simulink model "GasTurbine_PolyCompare_R3_Poly2FF"  (Simulink 9.2)
settings: Solver=ode4  StartTime=0.0  StopTime=MWS.in.SimTime  FixedStep=MWS.Solve.T  RelTol=1e-3  EnableMultiTasking=on
PreLoadFcn:
  | tmats_r3_poly2_setup;
values from neighbouring files (symbols this model uses):
  DOB = DOB0; DOB.gain=gains(j);DOB.mode=modes(j);DOB.fc=fcs(j)    [run_tmats_dob_study.m]
  MWS = tmats_gpt_setup()    [run_tmats_gpt.m]
undefined symbols (not defined in the file or in its folder): PTO, stripchar_TMATS, VF
libraries: Lib_Cntrl_FirstOrderSensor_TMATS x1, simulink x1, Lib_Turbo_Ambient_TMATS x1, Lib_Turbo_Burner_TMATS x1, Lib_Turbo_Compressor_TMATS x1, Lib_Turbo_Duct_TMATS x1, Lib_Turbo_Inlet_TMATS x1, Lib_Turbo_Nozzle_TMATS x1, Lib_Turbo_Shaft_TMATS x1, Lib_Turbo_Turbine_TMATS x1, Lib_Solve_IterNRSolverJC_TMATS x1, Lib_Solve_ModelSource_TMATS x1
Description:
  | 120 s speed-ramp and ambient cycle. See the cycle study usage notes.
settings Model: Creator=jwchapm2  LastModifiedBy=volka
settings DataIOCC: SignalLoggingSaveFormat=Dataset  SignalLoggingName=SimulationOutput
settings OptimizationCC: BlockReduction=off  DefaultParameterBehavior=Inlined  BufferReuse=off  ExpressionDepthLimit=2147483647
settings DebuggingCC: AlgebraicLoopMsg=error  SolverPrmCheckMsg=warning  FcnCallInpInsideContextMsg=error
settings GRTTargetCC: CombineOutputUpdateFcns=on  GRTInterface=off

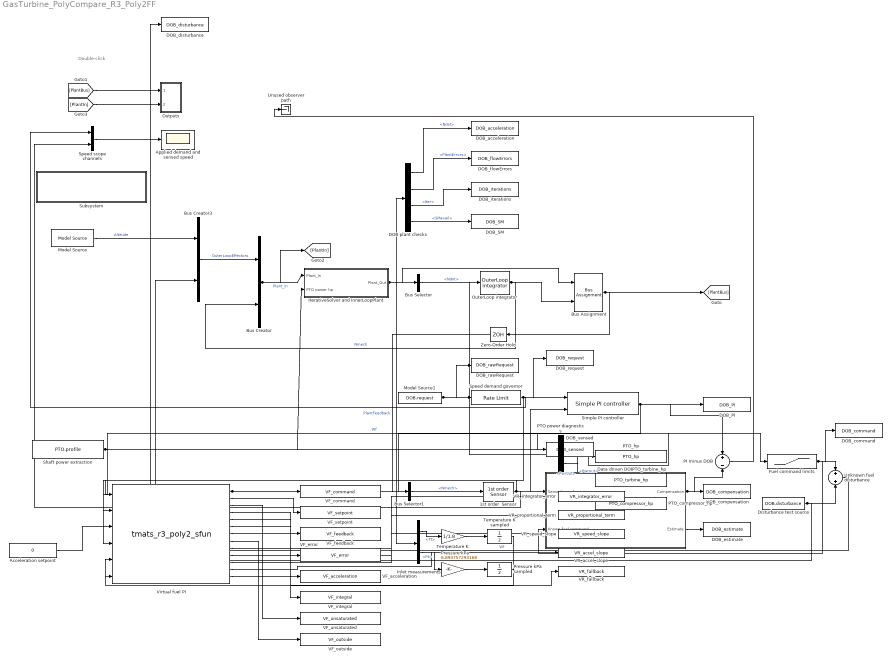
== system GasTurbine_PolyCompare_R3_Poly2FF ==
  note: Double-click
  1st order  Sensor : Lib_Cntrl_FirstOrderSensor_TMATS/1st order  Sensor  IC_M=MWS.Solve.N_IC  Sen_Max_M=20000  Sen_Min_M=0  Gain_M=1  Tau_M=0.05  GN_EN_M=off  GN_NST_M=MWS.Solve.T  GN_C_M=1  GN_MinNoise_M=0.3  F_Gain_M=1  F_Drift_M=0
  Acceleration setpoint : Constant  Value=0
  Applied demand and sensed speed : Scope
  Bus Assignment : BusAssignment  AssignedSignals=PlantBus.Nmech
  Bus Creator : BusCreator  Inputs=2
  Bus Creator3 : BusCreator  Inputs=2
  Bus Selector : BusSelector  OutputSignals=PlantBus.Ndot
  Bus Selector1 : BusSelector  OutputSignals=PlantBus.Nmech
  DOB plant checks : BusSelector  OutputSignals=PlantBus.Ndot,PlantErrors,PlantBus.Iter,PlantBus.C_Data.SMavail
  DOB_PI : ToWorkspace  VariableName=DOB_PI  SaveFormat=Timeseries  SampleTime=-1
  DOB_SM : ToWorkspace  VariableName=DOB_SM  SaveFormat=Timeseries  SampleTime=-1
  DOB_acceleration : ToWorkspace  VariableName=DOB_acceleration  SaveFormat=Timeseries  SampleTime=-1
  DOB_command : ToWorkspace  VariableName=DOB_command  SaveFormat=Timeseries  SampleTime=-1
  DOB_compensation : ToWorkspace  VariableName=DOB_compensation  SaveFormat=Timeseries  SampleTime=-1
  DOB_disturbance : ToWorkspace  VariableName=DOB_disturbance  SaveFormat=Timeseries  SampleTime=-1
  DOB_estimate : ToWorkspace  VariableName=DOB_estimate  SaveFormat=Timeseries  SampleTime=-1
  DOB_flowErrors : ToWorkspace  VariableName=DOB_flowErrors  SaveFormat=Timeseries  SampleTime=-1
  DOB_iterations : ToWorkspace  VariableName=DOB_iterations  SaveFormat=Timeseries  SampleTime=-1
  DOB_rawRequest : ToWorkspace  VariableName=DOB_rawRequest  SaveFormat=Timeseries  SampleTime=-1
  DOB_request : ToWorkspace  VariableName=DOB_request  SaveFormat=Timeseries  SampleTime=-1
  DOB_sensed : ToWorkspace  VariableName=DOB_sensed  SaveFormat=Timeseries  SampleTime=-1
  Data driven DOB : Subsystem
  Disturbance test source : FromWorkspace  VariableName=DOB.disturbance  SampleTime=DOB.Ts  Interpolate=off  OutputAfterFinalValue=Holding final value
  Fuel command limits : Saturate  UpperLimit=DOB.fuelMax  LowerLimit=DOB.fuelMin
  Inlet measurements : BusSelector  OutputSignals=PlantBus.s2.Tt,PlantBus.s2.Pt
  IterativeSolver and InnerLoopPlant : Subsystem
  Model Source : Lib_Solve_ModelSource_TMATS/Model Source  T_vec_M=MWS.in.t_vec  input_array_M=MWS.in.Alt
  Model Source1 : FromWorkspace  VariableName=DOB.request  SampleTime=DOB.Ts  Interpolate=off  OutputAfterFinalValue=Holding final value
  OuterLoop integrator : Lib_Solve_OuterLoopIntegrator_TMATS/OuterLoop integrator  OL_IC_M=MWS.Solve.N_IC
  Outputs : Subsystem
  PI minus DOB : Sum  Inputs=+-
  PTO power diagnostics : BusSelector  OutputSignals=PlantBus.T_Data.Pwrout,PlantBus.C_Data.Pwrout
  PTO_compressor_hp : ToWorkspace  VariableName=PTO_compressor_hp  SaveFormat=Timeseries  SampleTime=-1
  PTO_hp : ToWorkspace  VariableName=PTO_hp  SaveFormat=Timeseries  SampleTime=-1
  PTO_turbine_hp : ToWorkspace  VariableName=PTO_turbine_hp  SaveFormat=Timeseries  SampleTime=-1
  Pressure kPa : Gain  Gain=6.894757293168
  Pressure kPa sampled : UnitDelay  InitialCondition=99.298  SampleTime=VF.Ts
  Shaft power extraction : FromWorkspace  VariableName=PTO.profile  SampleTime=PTO.Ts  Interpolate=off  OutputAfterFinalValue=Holding final value
  Simple PI controller : Lib_Cntrl_SimplePIcontroller_TMATS/Simple PI controller  Kp_M=0.05/2  Ki_M=0.1/2  PI_IC_M=3
  Speed demand governor : RateLimiter  RisingSlewLimit=DOB.rate  FallingSlewLimit=-DOB.rate  SampleTimeMode=inherited  InitialCondition=10000
  Speed scope channels : Mux  Inputs=2
  Subsystem : Subsystem
      settings: OpenFcn=run('PlotDynData.m')
      mask Display: fprintf('Plot Outputs')
  Temperature K : Gain  Gain=1/1.8
  Temperature K sampled : UnitDelay  InitialCondition=288.15  SampleTime=VF.Ts
  Unknown fuel disturbance : Sum
  Unused observer path : Terminator
  VF_acceleration : ToWorkspace  VariableName=VF_acceleration  SaveFormat=Timeseries  SampleTime=-1
  VF_command : ToWorkspace  VariableName=VF_command  SaveFormat=Timeseries  SampleTime=-1
  VF_error : ToWorkspace  VariableName=VF_error  SaveFormat=Timeseries  SampleTime=-1
  VF_feedback : ToWorkspace  VariableName=VF_feedback  SaveFormat=Timeseries  SampleTime=-1
  VF_integral : ToWorkspace  VariableName=VF_integral  SaveFormat=Timeseries  SampleTime=-1
  VF_outside : ToWorkspace  VariableName=VF_outside  SaveFormat=Timeseries  SampleTime=-1
  VF_setpoint : ToWorkspace  VariableName=VF_setpoint  SaveFormat=Timeseries  SampleTime=-1
  VF_unsaturated : ToWorkspace  VariableName=VF_unsaturated  SaveFormat=Timeseries  SampleTime=-1
  VR_accel_slope : ToWorkspace  VariableName=VR_accel_slope  SaveFormat=Timeseries  SampleTime=-1
  VR_fallback : ToWorkspace  VariableName=VR_fallback  SaveFormat=Timeseries  SampleTime=-1
  VR_integrator_error : ToWorkspace  VariableName=VR_integrator_error  SaveFormat=Timeseries  SampleTime=-1
  VR_proportional_term : ToWorkspace  VariableName=VR_proportional_term  SaveFormat=Timeseries  SampleTime=-1
  VR_speed_slope : ToWorkspace  VariableName=VR_speed_slope  SaveFormat=Timeseries  SampleTime=-1
  Virtual fuel PI : M-S-Function  FunctionName=tmats_r3_poly2_sfun  Parameters=VF
  Zero-Order Hold : ZeroOrderHold  SampleTime=MWS.Solve.T
  wires:
  Data driven DOB/1(Compensation) -> PI minus DOB/2, DOB_compensation/1
  Bus Creator/1 -> [PlantIn], IterativeSolver and InnerLoopPlant/1(Plant_In)  "Plant_In"
  1st order  Sensor/1 -> Simple PI controller/2, Data driven DOB/1(Sensed speed), DOB_sensed/1, Speed scope channels/2, Virtual fuel PI/1
  OuterLoop integrator/1 -> Bus Creator/2, Bus Assignment/2  "Nmech"
  IterativeSolver and InnerLoopPlant/1(Plant_Out) -> Bus Assignment/1, Bus Selector/1, DOB plant checks/1, PTO power diagnostics/1, Inlet measurements/1
  Disturbance test source/1 -> Unknown fuel disturbance/2, DOB_disturbance/1
  Model Source1/1 -> Speed demand governor/1, DOB_rawRequest/1
  Fuel command limits/1 -> Unknown fuel disturbance/1, Data driven DOB/2(Known fuel command), DOB_command/1
  Simple PI controller/1 -> PI minus DOB/1, DOB_PI/1, Virtual fuel PI/4  "Wf"
  Speed demand governor/1 -> Simple PI controller/1, DOB_request/1, Speed scope channels/1, Virtual fuel PI/2
  Bus Assignment/1 -> [PlantBus], Zero-Order Hold/1
  Speed scope channels/1 -> Applied demand and sensed speed/1
  [PlantIn] -> Outputs/2(PlantIn)
  Data driven DOB/2(Estimate) -> DOB_estimate/1
  DOB plant checks/1 -> DOB_acceleration/1  "<Ndot>"
  DOB plant checks/2 -> DOB_flowErrors/1  "<PlantErrors>"
  Bus Creator3/1 -> Bus Creator/1  "OuterLoopEffectors"
  DOB plant checks/3 -> DOB_iterations/1  "<Iter>"
  DOB plant checks/4 -> DOB_SM/1  "<SMavail>"
  Unknown fuel disturbance/1 -> Bus Creator3/2  "Wf"
  [PlantBus] -> Outputs/1(PlantOut)
  Model Source/1 -> Bus Creator3/1  "Altitude"
  Bus Selector1/1 -> 1st order  Sensor/1  "<Nmech>"
  Bus Selector/1 -> OuterLoop integrator/1  "<Ndot>"
  Zero-Order Hold/1 -> Bus Selector1/1  "PlantFeedback"
  Shaft power extraction/1 -> IterativeSolver and InnerLoopPlant/2(PTO power hp), PTO_hp/1
  PTO power diagnostics/1 -> PTO_turbine_hp/1  "<Pwrout>"
  PTO power diagnostics/2 -> PTO_compressor_hp/1  "<Pwrout>"
  Acceleration setpoint/1 -> Virtual fuel PI/3
  PI minus DOB/1 -> Unused observer path/1
  Virtual fuel PI/1 -> Fuel command limits/1, VF_command/1
  Virtual fuel PI/2 -> VF_setpoint/1
  Virtual fuel PI/3 -> VF_feedback/1
  Virtual fuel PI/4 -> VF_error/1
  Virtual fuel PI/5 -> VF_acceleration/1
  Virtual fuel PI/6 -> VF_integral/1
  Virtual fuel PI/7 -> VF_unsaturated/1
  Virtual fuel PI/8 -> VF_outside/1
  Inlet measurements/1 -> Temperature K/1  "<Tt>"
  Temperature K/1 -> Temperature K sampled/1
  Temperature K sampled/1 -> Virtual fuel PI/5
  Inlet measurements/2 -> Pressure kPa/1  "<Pt>"
  Pressure kPa/1 -> Pressure kPa sampled/1
  Pressure kPa sampled/1 -> Virtual fuel PI/6
  Virtual fuel PI/9 -> VR_integrator_error/1
  Virtual fuel PI/10 -> VR_proportional_term/1
  Virtual fuel PI/11 -> VR_speed_slope/1
  Virtual fuel PI/12 -> VR_accel_slope/1
  Virtual fuel PI/13 -> VR_fallback/1

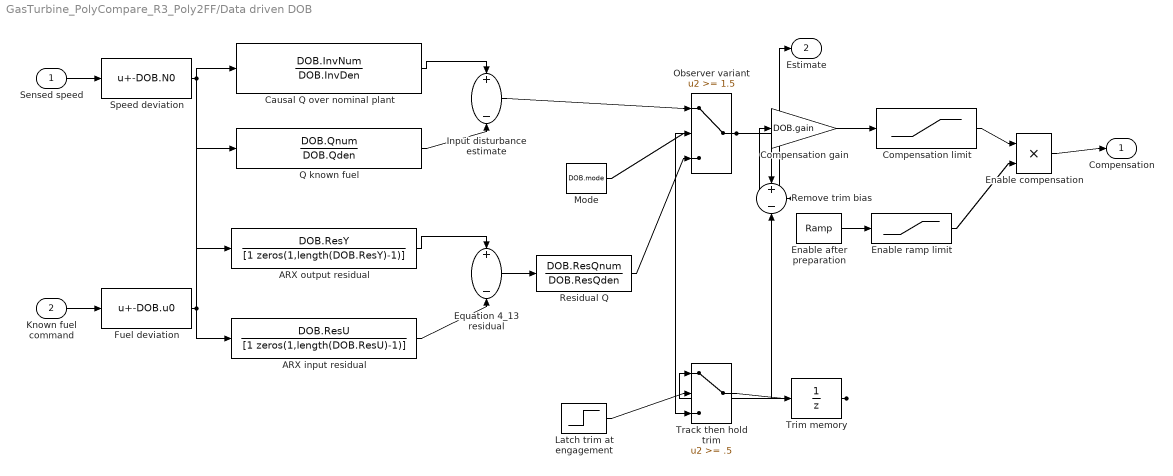
== system GasTurbine_PolyCompare_R3_Poly2FF/Data driven DOB ==
  Sensed speed : Inport
  Known fuel command : Inport  Port=2
  ARX input residual : DiscreteTransferFcn  Numerator=DOB.ResU  Denominator=[1 zeros(1,length(DOB.ResU)-1)]  SampleTime=DOB.Ts
  ARX output residual : DiscreteTransferFcn  Numerator=DOB.ResY  Denominator=[1 zeros(1,length(DOB.ResY)-1)]  SampleTime=DOB.Ts
  Causal Q over nominal plant : DiscreteTransferFcn  Numerator=DOB.InvNum  Denominator=DOB.InvDen  SampleTime=DOB.Ts
  Compensation gain : Gain  Gain=DOB.gain
  Compensation limit : Saturate  UpperLimit=DOB.compLimit  LowerLimit=-DOB.compLimit
  Enable after preparation : simulink/Sources/Ramp  slope=1/DOB.enableTime  start=DOB.start  InitialOutput=0
  Enable compensation : Product
  Enable ramp limit : Saturate  UpperLimit=1  LowerLimit=0
  Equation 4_13 residual : Sum  Inputs=+-
  Fuel deviation : Bias  Bias=-DOB.u0
  Input disturbance estimate : Sum  Inputs=+-
  Latch trim at engagement : Step  Time=DOB.start  SampleTime=DOB.Ts
  Mode : Constant  Value=DOB.mode
  Observer variant : Switch  Threshold=1.5
  Q known fuel : DiscreteTransferFcn  Numerator=DOB.Qnum  Denominator=DOB.Qden  SampleTime=DOB.Ts
  Remove trim bias : Sum  Inputs=+-
  Residual Q : DiscreteTransferFcn  Numerator=DOB.ResQnum  Denominator=DOB.ResQden  SampleTime=DOB.Ts
  Speed deviation : Bias  Bias=-DOB.N0
  Track then hold trim : Switch  Threshold=.5
  Trim memory : UnitDelay  SampleTime=DOB.Ts
  Compensation : Outport
  Estimate : Outport  Port=2
  wires:
  Sensed speed/1 -> Speed deviation/1
  Known fuel command/1 -> Fuel deviation/1
  Speed deviation/1 -> Causal Q over nominal plant/1, ARX output residual/1
  Fuel deviation/1 -> Q known fuel/1, ARX input residual/1
  Causal Q over nominal plant/1 -> Input disturbance estimate/1
  Q known fuel/1 -> Input disturbance estimate/2
  ARX output residual/1 -> Equation 4_13 residual/1
  ARX input residual/1 -> Equation 4_13 residual/2
  Equation 4_13 residual/1 -> Residual Q/1
  Input disturbance estimate/1 -> Observer variant/1
  Mode/1 -> Observer variant/2
  Residual Q/1 -> Observer variant/3
  Trim memory/1 -> Track then hold trim/1, Remove trim bias/2
  Latch trim at engagement/1 -> Track then hold trim/2
  Observer variant/1 -> Track then hold trim/3, Remove trim bias/1
  Track then hold trim/1 -> Trim memory/1
  Remove trim bias/1 -> Compensation gain/1, Estimate/1
  Compensation gain/1 -> Compensation limit/1
  Enable after preparation/1 -> Enable ramp limit/1
  Compensation limit/1 -> Enable compensation/1
  Enable ramp limit/1 -> Enable compensation/2
  Enable compensation/1 -> Compensation/1

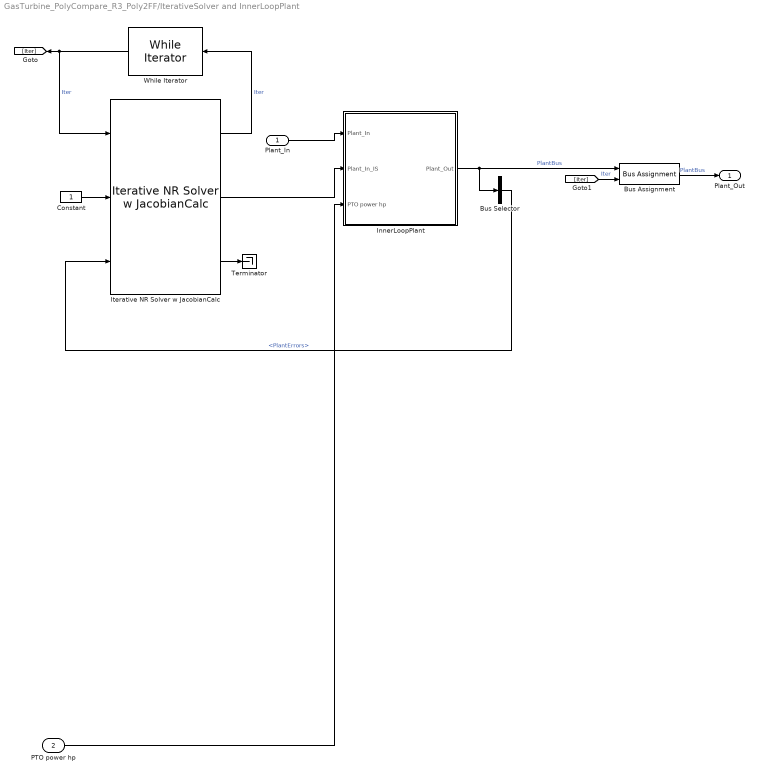
== system GasTurbine_PolyCompare_R3_Poly2FF/IterativeSolver and InnerLoopPlant ==
  Plant_In : Inport
  PTO power hp : Inport  Port=2
  Bus Assignment : BusAssignment  AssignedSignals=PlantBus.Iter
  Bus Selector : BusSelector  OutputSignals=PlantErrors
  Constant : Constant
  InnerLoopPlant : Subsystem
  Iterative NR Solver w JacobianCalc : Lib_Solve_IterNRSolverJC_TMATS/Iterative NR Solver w JacobianCalc  SJac_Per_M=MWS.Solve.J_Calc_Per  SNR_IC_M=MWS.Solve.NR_IC  SNR_DX_M=MWS.Solve.NR_dx  SNR_Mx_M=100000  SNR_Mn_M=0.0001  SJacobianAttempts_M=MWS.Solve.NR_Jac_Re  Cond_Limits_M=MWS.Solve.C_Lim
  Terminator : Terminator
  While Iterator : WhileIterator  MaxIters=MWS.Solve.Max_Iter  WhileBlockType=do-while  ShowIterationPort=on
  Plant_Out : Outport
  wires:
  Plant_In/1 -> InnerLoopPlant/1(Plant_In)
  Bus Selector/1 -> Iterative NR Solver w JacobianCalc/3  "<PlantErrors>"
  While Iterator/1 -> [Iter], Iterative NR Solver w JacobianCalc/1  "Iter"
  InnerLoopPlant/1(Plant_Out) -> Bus Assignment/1, Bus Selector/1  "PlantBus"
  Iterative NR Solver w JacobianCalc/2 -> InnerLoopPlant/2(Plant_In_IS)
  Iterative NR Solver w JacobianCalc/1 -> While Iterator/1  "Iter"
  Iterative NR Solver w JacobianCalc/3 -> Terminator/1
  Constant/1 -> Iterative NR Solver w JacobianCalc/2
  [Iter] -> Bus Assignment/2  "Iter"
  Bus Assignment/1 -> Plant_Out/1  "PlantBus"
  PTO power hp/1 -> InnerLoopPlant/3(PTO power hp)

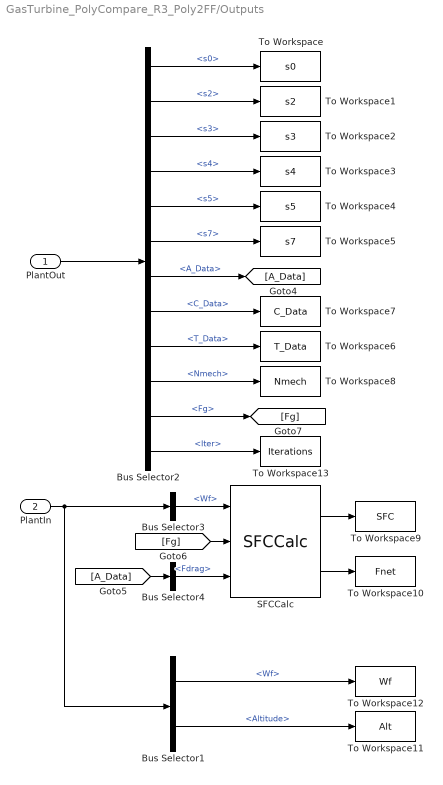
== system GasTurbine_PolyCompare_R3_Poly2FF/Outputs ==
  PlantOut : Inport
  PlantIn : Inport  Port=2
  Bus Selector1 : BusSelector  OutputSignals=OuterLoopEffectors.Wf,OuterLoopEffectors.Altitude
  Bus Selector2 : BusSelector  OutputSignals=PlantBus.s0,PlantBus.s2,PlantBus.s3,PlantBus.s4,PlantBus.s5,PlantBus.s7,PlantBus.A_Data,PlantBus.C_Data,PlantBus.T_Data,PlantBus.Nmech,PlantBus.Fg,PlantBus.Iter
  Bus Selector3 : BusSelector  OutputSignals=OuterLoopEffectors.Wf
  Bus Selector4 : BusSelector  OutputSignals=Fdrag
  SFCCalc : Lib_Turbo_SFCCalc_TMATS/SFCCalc
  To Workspace : ToWorkspace  VariableName=s0  SaveFormat=Timeseries  SampleTime=-1
  To Workspace1 : ToWorkspace  VariableName=s2  SaveFormat=Timeseries  SampleTime=-1
  To Workspace10 : ToWorkspace  VariableName=Fnet  SaveFormat=Timeseries  SampleTime=-1
  To Workspace11 : ToWorkspace  VariableName=Alt  SaveFormat=Timeseries  SampleTime=-1
  To Workspace12 : ToWorkspace  VariableName=Wf  SaveFormat=Timeseries  SampleTime=-1
  To Workspace13 : ToWorkspace  VariableName=Iterations  SaveFormat=Timeseries  SampleTime=-1
  To Workspace2 : ToWorkspace  VariableName=s3  SaveFormat=Timeseries  SampleTime=-1
  To Workspace3 : ToWorkspace  VariableName=s4  SaveFormat=Timeseries  SampleTime=-1
  To Workspace4 : ToWorkspace  VariableName=s5  SaveFormat=Timeseries  SampleTime=-1
  To Workspace5 : ToWorkspace  VariableName=s7  SaveFormat=Timeseries  SampleTime=-1
  To Workspace6 : ToWorkspace  VariableName=T_Data  SaveFormat=Timeseries  SampleTime=-1
  To Workspace7 : ToWorkspace  VariableName=C_Data  SaveFormat=Timeseries  SampleTime=-1
  To Workspace8 : ToWorkspace  VariableName=Nmech  SaveFormat=Timeseries  SampleTime=-1
  To Workspace9 : ToWorkspace  VariableName=SFC  SaveFormat=Timeseries  SampleTime=-1
  wires:
  SFCCalc/2 -> To Workspace10/1
  Bus Selector2/5 -> To Workspace4/1  "<s5>"
  SFCCalc/1 -> To Workspace9/1
  Bus Selector3/1 -> SFCCalc/1  "<Wf>"
  Bus Selector2/6 -> To Workspace5/1  "<s7>"
  Bus Selector2/11 -> [Fg]  "<Fg>"
  Bus Selector4/1 -> SFCCalc/3  "<Fdrag>"
  Bus Selector2/10 -> To Workspace8/1  "<Nmech>"
  Bus Selector2/1 -> To Workspace/1  "<s0>"
  Bus Selector2/3 -> To Workspace2/1  "<s3>"
  Bus Selector2/8 -> To Workspace7/1  "<C_Data>"
  Bus Selector2/9 -> To Workspace6/1  "<T_Data>"
  Bus Selector2/7 -> [A_Data]  "<A_Data>"
  PlantOut/1 -> Bus Selector2/1
  [Fg] -> SFCCalc/2
  Bus Selector2/2 -> To Workspace1/1  "<s2>"
  Bus Selector2/4 -> To Workspace3/1  "<s4>"
  PlantIn/1 -> Bus Selector1/1, Bus Selector3/1
  [A_Data] -> Bus Selector4/1
  Bus Selector1/1 -> To Workspace12/1  "<Wf>"
  Bus Selector1/2 -> To Workspace11/1  "<Altitude>"
  Bus Selector2/12 -> To Workspace13/1  "<Iter>"

== system GasTurbine_PolyCompare_R3_Poly2FF/Subsystem ==

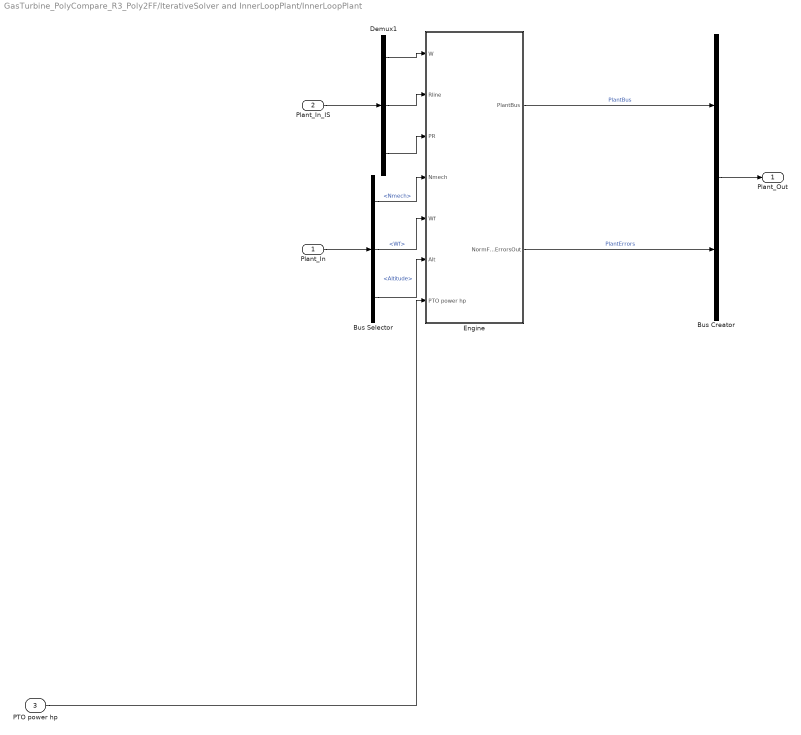
== system GasTurbine_PolyCompare_R3_Poly2FF/IterativeSolver and InnerLoopPlant/InnerLoopPlant ==
  Plant_In : Inport
  Plant_In_IS : Inport  Port=2
  PTO power hp : Inport  Port=3
  Bus Selector : BusSelector  OutputSignals=Nmech,OuterLoopEffectors.Wf,OuterLoopEffectors.Altitude
  Bus Creator : BusCreator  Inputs=2
  Demux1 : Demux  Outputs=3
  Engine : Subsystem
  Plant_Out : Outport
  wires:
  Engine/1(PlantBus) -> Bus Creator/1  "PlantBus"
  Engine/2(NormFlowErrorsOut) -> Bus Creator/2  "PlantErrors"
  Bus Creator/1 -> Plant_Out/1
  Bus Selector/2 -> Engine/5(Wf)  "<Wf>"
  Bus Selector/1 -> Engine/4(Nmech)  "<Nmech>"
  Bus Selector/3 -> Engine/6(Alt)  "<Altitude>"
  Demux1/1 -> Engine/1(W)
  Demux1/2 -> Engine/2(Rline)
  Demux1/3 -> Engine/3(PR)
  Plant_In/1 -> Bus Selector/1
  Plant_In_IS/1 -> Demux1/1
  PTO power hp/1 -> Engine/7(PTO power hp)

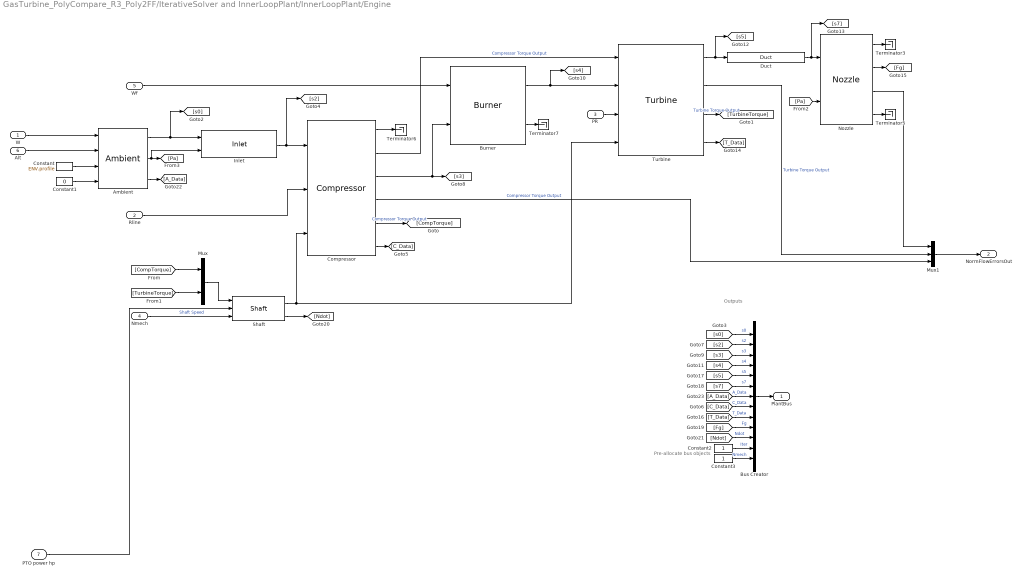
== system GasTurbine_PolyCompare_R3_Poly2FF/IterativeSolver and InnerLoopPlant/InnerLoopPlant/Engine ==
  note: Pre-allocate bus objects
  note: Outputs
  W : Inport
  Rline : Inport  Port=2
  PR : Inport  Port=3
  Nmech : Inport  Port=4
  Wf : Inport  Port=5
  Alt : Inport  Port=6
  PTO power hp : Inport  Port=7
  Ambient : Lib_Turbo_Ambient_TMATS/Ambient  X_A_AltVec_M=5000*[-1 0 1 2 3 4 5 6 7 8 9 10 12 14 16]  T_A_TsVec_M=[536.51 518.67 500.84 483.03 465.22 447.41 429.62 411.84 394.06 389.97 389.97 389.97 389.97 392.25 397.69]  T_A_PsVec_M=[17.554 14.696 12.228 10.108 8.297 6.759 5.461 4.373 3.468 2.73 2.149 1.692 1.049 0.651 0.406]  AFARc_M=0  X_A_FARVec_M=[0; 0.0050; 0.0100; 0.0150; 0.0200; 0.0250; 0.0300]  T_A_RtArray_M="[0.0686;    0.0686;    0.0686;    0.0686;    0.0686;    0.0686;    0.0686]"  Y_A_TVec_M=[300 10000]  T_A_gammaArray_M=[ 1.4 1.4 1.4 1.4 1.4 1.4 1.4; 1.4 1.4 1.4 1.4 1.4 1.4 1.4]
  Burner : Lib_Turbo_Burner_TMATS/Burner  LHVEn_M=on  LHV_M=MWS.Burner.LHV  Eff_M=1  hFuel_M=-1200  dPnormBurner_M=MWS.Burner.dP
  Bus Creator : BusCreator  Inputs=13
  Compressor : Lib_Turbo_Compressor_TMATS/Compressor  X_C_RlineVec_M=MWS.HPC.RlineVec  Z_C_AlphaVec_M=1  Y_C_Map_NcVec_M=MWS.HPC.NcVec  T_C_Map_WcArray_M=MWS.HPC.WcArray  T_C_Map_PRArray_M=MWS.HPC.PRArray  T_C_Map_EffArray_M=MWS.HPC.EffArray  s_C_Nc_M=MWS.HPC.s_Nc  s_C_Wc_M=MWS.HPC.s_Wc  s_C_PR_M=MWS.HPC.s_PR  s_C_Eff_M=MWS.HPC.s_eff  SL_M=off  Scale_M=none  CBLDEN_M=off  C_CBD_M=0  C_CBFht_M=0.5  C_CBFPt_M=0.5  FBLDEN_M=off  C_FBD_M=0  C_BFht_M=0.5  C_BFPt_M=0.5  DefSMEn_M=off  SMNEn_M=off  SRline_M=1  X_C_Map_WcSurgeVec_M=MWS.HPC.WcMapSurge  T_C_Map_PRSurgeVec_M=MWS.HPC.PRMapSurge  iDesign_M=2  NcDes_M=10000  EffDes_M=0.85  PRDes_M=20  RlineDes_M=2  FVar_M=strcat('iDes_',stripchar_TMATS(gcb),'.bin')  BlkNm_M=double(gcb)  HP_M=off
  Constant : FromWorkspace  VariableName=ENV.profile  OutputAfterFinalValue=Holding final value
  Constant1 : Constant  Value=0
  Constant2 : Constant  OutDataTypeStr=int32
  Constant3 : Constant
  Duct : Lib_Turbo_Duct_TMATS/Duct  dP_M=MWS.Duct.dP
  Inlet : Lib_Turbo_Inlet_TMATS/Inlet  eRambase_M=MWS.Inlet.eRambase  X_eRamVec_M=[0 3]  T_eRamtbl_M=[1 1]
  Mux : Mux  Inputs=2
  Mux1 : Mux  Inputs=3
  Nozzle : Lib_Turbo_Nozzle_TMATS/Nozzle  SWType_M=Convergent  N_TArea_M=MWS.Noz.ATh  N_EArea_M=110.7  N_FL_M=MWS.Noz.LossPerc  X_N_TtVec2_M=MWS.Noz.TtVec  T_N_TGArray_M=MWS.Noz.TGArray  X_N_PEQPaVec_M=MWS.Noz.PeQPaVec  T_N_CdThArray_M=MWS.Noz.CdThArray  T_N_CvArray_M=MWS.Noz.CvArray  CfgEn_M=off  T_N_CfgArray_M=[1 1]  X_N_FARVec_M=MWS.Noz.FARVec  T_N_RtArray_M=MWS.Noz.RArray  Y_N_TtVec_M=MWS.Noz.TtVec  T_N_MAP_gammaArray_M=MWS.Noz.GArray  iDesign_M=2  WDes_M=100  FVar_M=strcat('iDes_',stripchar_TMATS(gcb),'.bin')
  Shaft : Lib_Turbo_Shaft_TMATS/Shaft  Shaft_Inertia_M=MWS.Shaft.N_I
  Terminator{3,5..7} (4 alike) : Terminator
  Turbine : Lib_Turbo_Turbine_TMATS/Turbine  X_T_Map_PRVec_M=MWS.HPT.PRVec  Y_T_Map_NcVec_M=MWS.HPT.NcVec  T_T_Map_WcArray_M=MWS.HPT.WcArray  T_T_Map_EffArray_M=MWS.HPT.EffArray  s_T_Nc_M=MWS.HPT.s_Nc  s_T_Wc_M=MWS.HPT.s_Wc  s_T_PR_M=MWS.HPT.s_PR  s_T_Eff_M=MWS.HPT.s_eff  ConfigNPSS_M=0  Scale_M=none  CFlwEn_M=off  T_CoolFlwPos_M=0  iDesign_M=2  NcDes_M=100  EffDes_M=0.9200  PRDes_M=5  NDes_M=10000  FVar_M=strcat('iDes_',stripchar_TMATS(gcb),'.bin')  BlkNm_M=double(gcb)  HP_M=off
  PlantBus : Outport
  NormFlowErrorsOut : Outport  Port=2
  wires:
  Compressor/6 -> [C_Data]
  Ambient/1 -> [s0], Inlet/1
  Duct/1 -> [s7], Nozzle/1
  Ambient/3 -> [A_Data]
  Ambient/2 -> [Pa], Inlet/2
  Constant1/1 -> Ambient/4
  W/1 -> Ambient/1
  Nozzle/2 -> [Fg]
  Compressor/2 -> Turbine/1  "Compressor Torque Output"
  Compressor/1 -> Terminator6/1
  Shaft/1 -> Compressor/3, Turbine/4
  [TurbineTorque] -> Mux/2
  [CompTorque] -> Mux/1
  Turbine/3 -> [TurbineTorque]  "Turbine Torque Output"
  Compressor/5 -> [CompTorque]  "Compressor Torque Output"
  Mux/1 -> Shaft/1
  Shaft/2 -> [Ndot]
  Nmech/1 -> Shaft/3  "Shaft Speed"
  Inlet/1 -> [s2], Compressor/1
  Alt/1 -> Ambient/2
  Compressor/4 -> Mux1/3  "Compressor Torque Output"
  Turbine/2 -> Mux1/2  "Turbine Torque Output"
  Nozzle/4 -> Terminator5/1
  Nozzle/3 -> Mux1/1
  Nozzle/1 -> Terminator3/1
  Turbine/4 -> [T_Data]
  Mux1/1 -> NormFlowErrorsOut/1
  Rline/1 -> Compressor/2
  PR/1 -> Turbine/3
  Turbine/1 -> [s5], Duct/1
  Burner/1 -> [s4], Turbine/2
  [Pa] -> Nozzle/2
  Burner/2 -> Terminator7/1
  Wf/1 -> Burner/1
  Compressor/3 -> [s3], Burner/2
  [s0] -> Bus Creator/1  "s0"
  [s2] -> Bus Creator/2  "s2"
  [s3] -> Bus Creator/3  "s3"
  [s4] -> Bus Creator/4  "s4"
  [s5] -> Bus Creator/5  "s5"
  [s7] -> Bus Creator/6  "s7"
  [C_Data] -> Bus Creator/8  "C_Data"
  [T_Data] -> Bus Creator/9  "T_Data"
  [Fg] -> Bus Creator/10  "Fg"
  [Ndot] -> Bus Creator/11  "Ndot"
  Bus Creator/1 -> PlantBus/1
  [A_Data] -> Bus Creator/7  "A_Data"
  Constant2/1 -> Bus Creator/12  "Iter"
  Constant3/1 -> Bus Creator/13  "Nmech"
  PTO power hp/1 -> Shaft/2
  Constant/1 -> Ambient/3
